simulink model "lqi8_continuo"  (R2025b)
settings: Solver=VariableStepAuto  StartTime=0.0  StopTime=10  RelTol=1e-3
values from neighbouring files (symbols this model uses):
  K = [8.61388977208e-09 -3.23938755891e-11 27.1624608635 1.22408347835e-11 5.15548702544e-09 -26.9052309444 4.91703547324e-11 2.27757364143e-13 56.1282376315 -9.6103215742e-14 8.73666069887e-14 -5.56559839576e-15 ... (64 elements, 4x16)]    [parametros_LQI.mat]
undefined symbols (not defined in the file or in its folder): A, B, C, L
libraries: simulink x1
settings Model: Creator=rel  LastModifiedBy=rel

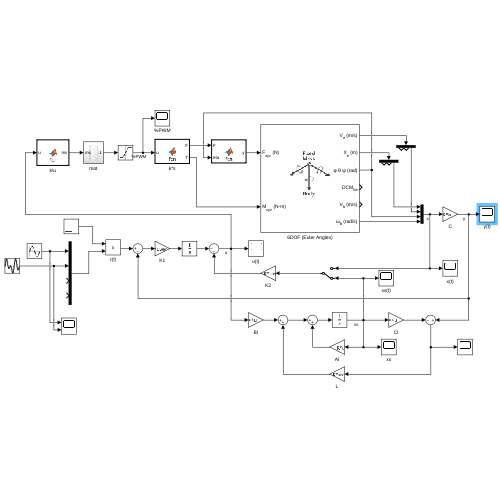
[thumbnail: Simulink's stored preview of the top-level diagram]
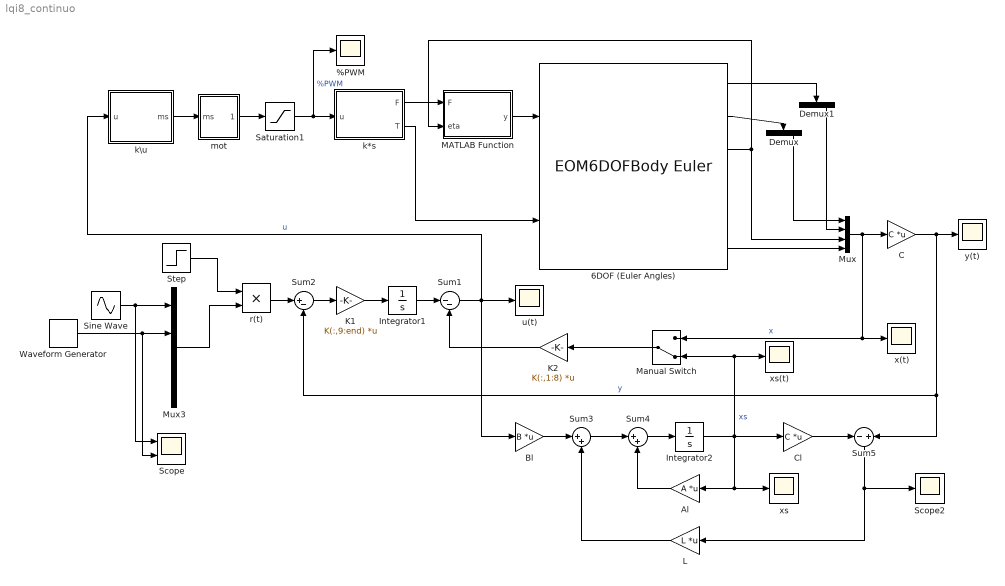
== system lqi8_continuo ==
  %PWM : Scope
      settings: ActiveDisplayYMinimum=-1  ActiveDisplayYMaximum=1  DataLoggingVariableName=ScopeData4
  6DOF (Euler Angles) : EOM6DOFBodyEuler  mass_0=1.6  inertia=diag([0.021915027 0.022124548 0.042349865])
  Al : Gain  Gain=A  Multiplication=Matrix(K*u)
  Bl : Gain  Gain=B  Multiplication=Matrix(K*u)
  C : Gain  Gain=C  Multiplication=Matrix(K*u)
  Cl : Gain  Gain=C  Multiplication=Matrix(K*u)
  Demux : Demux  Outputs=3
  Demux1 : Demux  Outputs=3
  Integrator1 : Integrator
  Integrator2 : Integrator
  K1 : Gain  Gain=K(:,9:end)  Multiplication=Matrix(K*u) (u vector)
  K2 : Gain  Gain=K(:,1:8)  Multiplication=Matrix(K*u) (u vector)
  L : Gain  Gain=L  Multiplication=Matrix(K*u) (u vector)
  MATLAB Function : MATLAB Function  TreatAsAtomicUnit=on
  Manual Switch : ManualSwitch  CurrentSetting=0
  Mux : Mux
  Mux3 : Mux
  Saturation1 : Saturate  UpperLimit=1  LowerLimit=0
  Scope : Scope  NumInputPorts=2
      settings: ActiveDisplayYMinimum=-0.41227021130108987  ActiveDisplayYMaximum=1.7124682918159155  DataLoggingVariableName=ScopeData2
  Scope2 : Scope
      settings: ActiveDisplayYMinimum=-1  ActiveDisplayYMaximum=1  DataLoggingVariableName=ScopeData6
  Sine Wave : Sin  Amplitude=0.5  Bias=1  Frequency=5  SampleTime=0
  Step : Step  SampleTime=0
  Sum1 : Sum  Inputs=|--
  Sum2 : Sum  Inputs=|+-
  Sum3 : Sum  Inputs=|++
  Sum4 : Sum  Inputs=|++
  Sum5 : Sum  Inputs=-|+
  Waveform Generator : simulink/Sources/Waveform Generator  OutMin=[]  OutMax=[]  OutDataTypeStr=double  SelectedSignal=1  Signals=sin(0.2, 3, 1)#sin(0.2,8,1)  BlockNames=MultiportSwitch_86f2a32215fc4c1#MultiportSwitch_93f6231ef87447f  SampleTime=0.1
  k*s : MATLAB Function  TreatAsAtomicUnit=on
  k\u : MATLAB Function  TreatAsAtomicUnit=on
  mot : Subsystem
  r(t) : Product
  u(t) : Scope
      settings: ActiveDisplayYMinimum=-2.80318631668736  ActiveDisplayYMaximum=24.946088998582049
  x(t) : Scope
      settings: ActiveDisplayYMinimum=-0.8612526795618034  ActiveDisplayYMaximum=1.557087851784861  DataLoggingVariableName=ScopeData3
  xs : Scope
      settings: ActiveDisplayYMinimum=-1.2850581790493911  ActiveDisplayYMaximum=2.2978317930607965  DataLoggingVariableName=ScopeData5
  xs(t) : Scope
      settings: ActiveDisplayYMinimum=-1  ActiveDisplayYMaximum=1  DataLoggingVariableName=ScopeData7
  y(t) : Scope
      settings: ActiveDisplayYMinimum=-0.31926975162060495  ActiveDisplayYMaximum=1.2715507253602278
  wires:
  C/1 -> y(t)/1, Sum2/2, Sum5/2  "y"
  Step/1 -> r(t)/1
  r(t)/1 -> Sum2/1
  K2/1 -> Sum1/2
  K1/1 -> Integrator1/1
  Sum2/1 -> K1/1
  Integrator1/1 -> Sum1/1
  6DOF (Euler Angles)/2 -> Demux/1
  6DOF (Euler Angles)/3 -> Mux/3, MATLAB Function/2(eta)
  6DOF (Euler Angles)/1 -> Demux1/1
  mot/1(Out1) -> Saturation1/1
  k\u/1(ms) -> mot/1(ms)
  Saturation1/1 -> %PWM/1, k*s/1(u)  "%PWM"
  k*s/2(T) -> 6DOF (Euler Angles)/2
  Mux3/1 -> r(t)/2
  Sine Wave/1 -> Scope/1, Mux3/1
  Waveform Generator/1 -> Mux3/2, Scope/2
  k*s/1(F) -> MATLAB Function/1(F)
  MATLAB Function/1(y) -> 6DOF (Euler Angles)/1
  Bl/1 -> Sum3/1
  Sum3/1 -> Sum4/1
  Sum4/1 -> Integrator2/1
  Integrator2/1 -> xs(t)/1, Manual Switch/2, Cl/1, xs/1, Al/1  "xs"
  Cl/1 -> Sum5/1
  Al/1 -> Sum4/2
  L/1 -> Sum3/2
  Sum5/1 -> L/1, Scope2/1
  Sum1/1 -> u(t)/1, k\u/1(u), Bl/1  "u"
  Demux/3 -> Mux/1
  Demux1/3 -> Mux/2
  6DOF (Euler Angles)/6 -> Mux/4
  Mux/1 -> x(t)/1, Manual Switch/1, C/1  "x"
  Manual Switch/1 -> K2/1

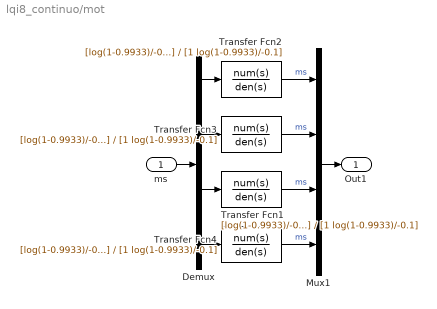
== system lqi8_continuo/mot ==
  ms : Inport
  Demux : Demux
  Mux1 : Mux
  Transfer Fcn{1..4} (4 alike) : TransferFcn  Numerator=[log(1-0.9933)/-0.1]  Denominator=[1 log(1-0.9933)/-0.1]
  Out1 : Outport
  wires:
  Transfer Fcn3/1 -> Mux1/2  "ms"
  Transfer Fcn1/1 -> Mux1/3  "ms"
  Demux/3 -> Transfer Fcn1/1
  Transfer Fcn4/1 -> Mux1/4  "ms"
  Demux/4 -> Transfer Fcn4/1
  Mux1/1 -> Out1/1
  Transfer Fcn2/1 -> Mux1/1  "ms"
  Demux/2 -> Transfer Fcn3/1
  Demux/1 -> Transfer Fcn2/1
  ms/1 -> Demux/1

== matlab function lqi8_continuo/k\u ==
  data: u input; ms output
function ms = fcn(u)
% L = 0.0080;
% kF = 0.1600*9.81;
% kM = 0.0086;
L = 0.268554;
kF = 0.7*9.81;
kM = 0.2;
A = [kF kF kF kF; -L*kF -L*kF L*kF L*kF; L*kF -L*kF -L*kF L*kF; -kM kM -kM kM];
ms = A\[u(1); u(2:end)];

== matlab function lqi8_continuo/MATLAB Function ==
  data: F input; y output; eta input
function y = fcn(F, eta)
phi = eta(1);
theta = eta(2);
psi = eta(3);
y = [0;0;-1.6*9.81] + [sin(theta)*cos(psi) + sin(phi)*cos(theta)*sin(psi); ...
                    sin(theta)*sin(psi) - sin(phi)*cos(theta)*cos(psi); ...
                    cos(phi)*cos(theta)]*F;

== matlab function lqi8_continuo/k*s ==
  data: u input; F output; T output
function [F, T] = fcn(u)
% L = 0.0080;
% kF = 0.1600*9.81;
% kM = 0.0086;
L = 0.268554;
kF = 0.7*9.81;
kM = 0.2;
A = [kF kF kF kF; -L*kF -L*kF L*kF L*kF; L*kF -L*kF -L*kF L*kF; -kM kM -kM kM];
y = A*u;
F = y(1);
T = y(2:end);
